simulink model "RNEDynamicsTask"  (R2022b)
settings: Solver=ode45  StartTime=0.0  StopTime=tSim  RelTol=1e-7
values from neighbouring files (symbols this model uses):
  freq = 2*pi/tSim * numOscillations    (= 0.314159265359)    [main.m]    (also in mainJoint.m = 0.209439510239)
  KdInner = 20 * eye(6)    [main.m]    (also in mainJoint.m = 40 * eye(6))
  KpInner = 4 * eye(6)    [main.m]    (also in mainJoint.m)
  maxSinAmount = 100    [main.m]    (also in mainJoint.m = 80)
  Robot = SerialLink(L)    [main.m]    (also in mainJoint.m)
  theta0Per = theta0    [main.m]
  tSim = 30    [main.m]    (also in mainJoint.m)
  xDesIC = [state0',ori0']'    [main.m]
  xIC = [state0Per',ori0Per']'    [main.m]
undefined symbols (not defined in the file or in its folder): calcTorques, Jacobian0_analytical, manipulatorPlant, tAccel2jAccel
settings Model: Creator=Hunter  LastModifiedBy=Hunter
settings SolverCC: MaxConsecutiveMinStep=3

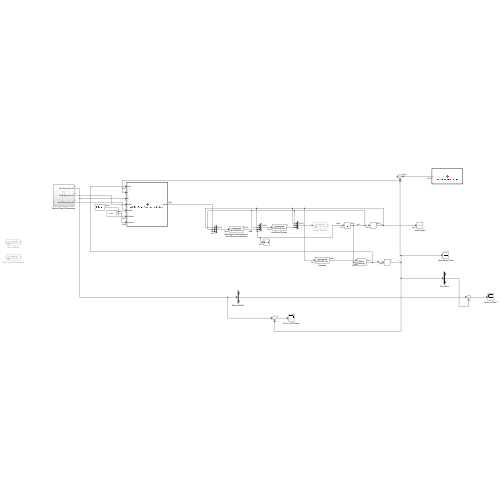
[thumbnail: Simulink's stored preview of the top-level diagram]
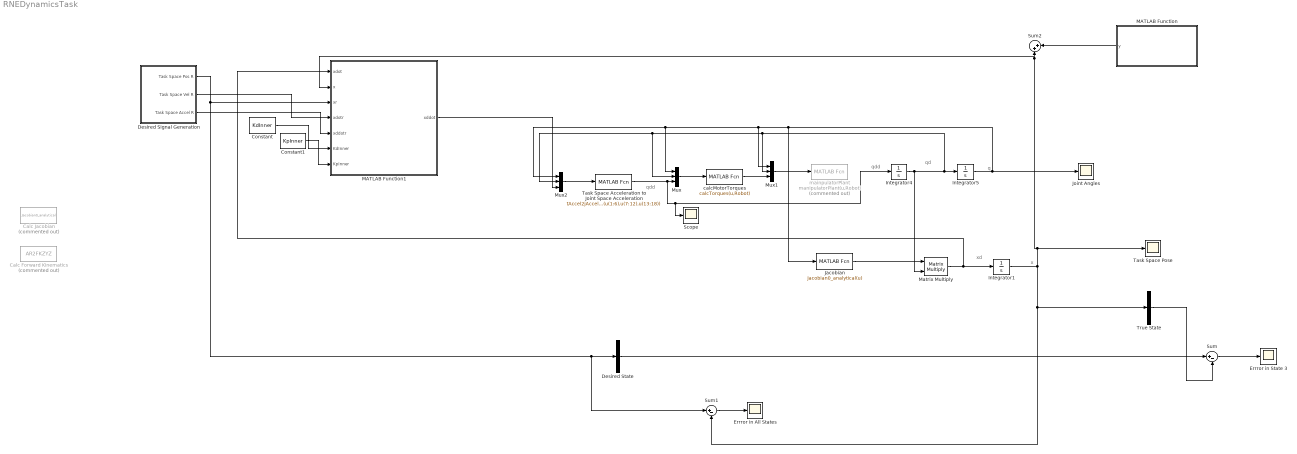
== system RNEDynamicsTask ==
  note: qdd
  note: x
  note: xd
  note: q
  note: qd
  note: qdd
  Calc Forward Kinematics : MATLABFcn  Commented=on  MATLABFcn=AR2FKZYZ
  Calc Jacobian : MATLABFcn  Commented=on  MATLABFcn=Jacobian0_analytical
  Constant : Constant  Value=KdInner
  Constant1 : Constant  Value=KpInner
  Desired Signal Generation : Subsystem
  Desired State : Demux  Outputs=[2 1 3]
  Errror in All States : Scope
  Errror in State 3 : Scope
  Integrator1 : Integrator  InitialCondition=xIC
  Integrator4 : Integrator  InitialCondition=[0 0 0 0 0 0]'
  Integrator5 : Integrator  InitialCondition=theta0Per'
  Jacobian : MATLABFcn  MATLABFcn=Jacobian0_analytical(u)  Output1D=off
  Joint Angles : Scope
  MATLAB Function : MATLAB Function  TreatAsAtomicUnit=on
  MATLAB Function1 : MATLAB Function  TreatAsAtomicUnit=on
  Matrix Multiply : Product  Multiplication=Matrix(*)
  Mux : Mux  Inputs=3
  Mux1 : Mux  Inputs=3
  Mux2 : Mux  Inputs=3
  Scope : Scope
  Sum : Sum  Inputs=|+-
  Sum1 : Sum  Inputs=|+-
  Sum2 : Sum  Inputs=|++
  Task Space Acceleration to Joint Space Acceleration : MATLABFcn  MATLABFcn=tAccel2jAccel(u(1:6),u(7:12),u(13:18))  Output1D=off
  Task Space Pose : Scope
  True State : Demux  Outputs=[2 1 3]
  calcMotorTorques : MATLABFcn  MATLABFcn=calcTorques(u,Robot)  OutputDimensions=6  Output1D=off
  mainpulatorPlant : MATLABFcn  Commented=on  MATLABFcn=manipulatorPlant(u,Robot)
  wires:
  Desired Signal Generation/1(Task Space Pos R) -> MATLAB Function1/3(xr), Desired State/1, Sum1/1
  Constant/1 -> MATLAB Function1/6(KdInner)
  Constant1/1 -> MATLAB Function1/7(KpInner)
  MATLAB Function1/1(xddot) -> Mux2/3
  Mux/1 -> calcMotorTorques/1
  Task Space Acceleration to Joint Space Acceleration/1 -> Scope/1, Integrator4/1, Mux/3
  calcMotorTorques/1 -> Mux1/3
  Mux1/1 -> mainpulatorPlant/1
  Integrator4/1 -> Integrator5/1, Mux1/2, Mux/2, Mux2/2, Matrix Multiply/2
  Integrator5/1 -> Jacobian/1, Mux1/1, Mux/1, Mux2/1, Joint Angles/1
  Jacobian/1 -> Matrix Multiply/1
  Matrix Multiply/1 -> Integrator1/1, MATLAB Function1/1(xdot)
  Integrator1/1 -> Task Space Pose/1, MATLAB Function1/2(x), Sum2/2, True State/1, Sum1/2
  Mux2/1 -> Task Space Acceleration to Joint Space Acceleration/1
  Desired State/2 -> Sum/1
  True State/2 -> Sum/2
  Desired Signal Generation/2(Task Space Vel R) -> MATLAB Function1/4(xdotr)
  Desired Signal Generation/3(Task Space Accel R) -> MATLAB Function1/5(xddotr)
  Sum/1 -> Errror in State 3/1
  Sum1/1 -> Errror in All States/1
  MATLAB Function/1(y) -> Sum2/1

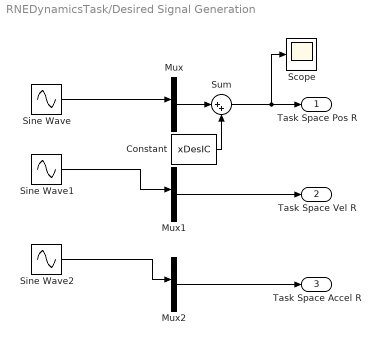
== system RNEDynamicsTask/Desired Signal Generation ==
  Constant : Constant  Value=xDesIC
  Mux : Mux  Inputs=6
  Mux1 : Mux  Inputs=6
  Mux2 : Mux  Inputs=6
  Scope : Scope
  Sine Wave : Sin  Amplitude=maxSinAmount  Frequency=freq  SampleTime=0
  Sine Wave1 : Sin  Amplitude=maxSinAmount * (2 * pi / tSim)  Frequency=freq  Phase=pi/2  SampleTime=0
  Sine Wave2 : Sin  Amplitude=-maxSinAmount * (2 * pi / tSim)^2  Frequency=freq  SampleTime=0
  Sum : Sum  Inputs=|++
  Task Space Pos R : Outport
  Task Space Vel R : Outport  Port=2
  Task Space Accel R : Outport  Port=3
  wires:
  Sine Wave/1 -> Mux/3
  Sine Wave1/1 -> Mux1/3
  Sine Wave2/1 -> Mux2/3
  Mux2/1 -> Task Space Accel R/1
  Mux1/1 -> Task Space Vel R/1
  Mux/1 -> Sum/1
  Constant/1 -> Sum/2
  Sum/1 -> Scope/1, Task Space Pos R/1

== matlab function RNEDynamicsTask/MATLAB Function1 ==
  data: xdot input; xddot output; x input; xr input; xdotr input; xddotr input; KdInner input; KpInner input
function xddot = calcTaskSpaceAccelerationController(xdot,x,xr,xdotr,xddotr,KdInner,KpInner)

xddot = (xddotr - KdInner * (xdot-xdotr) - KpInner * (x - xr));

== matlab function RNEDynamicsTask/MATLAB Function ==
  data: y output
function y = gaussianWhiteNoiseGen()

y = wgn(6,1,-10);
